simulink model "MySusp_TopMount_RTW"  (Simulink 10.3)
settings: Solver=ode1  StartTime=0.0  StopTime=inf  FixedStep=0.001  RelTol=1e-3
PreLoadFcn:
  | vehicle = 'Car'; if ~length(which('cmself')), cmenv; end
  | MySusp_TopMount_RTW_params
InitFcn:
  | vehicle = 'Car'; if ~length(which('cmself')), cmenv; end
  | MySusp_TopMount_RTW_bus
undefined symbols (not defined in the file or in its folder): cTM, dTM, mTM
Description:
  | CarMaker Plug-in Model Target
settings Model: Creator=ml  ModifiedByFormat=IPG  LastModifiedBy=IPG  MultithreadedSim=on
settings DataIOCC: SaveFormat=Dataset  SignalLoggingSaveFormat=Dataset  ReturnWorkspaceOutputs=on
settings OptimizationCC: ExpressionDepthLimit=128  LifeSpan=auto
settings DebuggingCC: UnderspecifiedInitializationDetection=Simplified  MergeDetectMultiDrivingBlocksExec=error  FcnCallInpInsideContextMsg=error  StateNameClashWarn=none  SFUnexpectedBacktrackingDiag=error  SFNoUnconditionalDefaultTransitionDiag=error  SFExecutionAtInitializationDiag=warning  ArithmeticOperatorsInVariantConditions=error
settings HardwareCC: ProdBitPerPointer=64  ProdBitPerSizeT=64  ProdBitPerPtrDiffT=64  ProdLargestAtomicFloat=Float  ProdIntDivRoundTo=Zero  ProdEndianess=LittleEndian  ProdWordSize=64  ProdHWDeviceType=Intel->x86-64 (Windows64)
settings ModelReferenceCC: PropagateSignalLabelsOutOfModel=on
settings SFSimCC: SimUseLocalCustomCode=on  CustomCodeUndefinedFunction=FilterOut
settings RTWCC: Description=CarMaker Plug-in Model Target  SystemTargetFile=CarMaker.tlc  TemplateMakefile=CarMaker_unix-win64.tmf  RTWUseLocalCustomCode=on
settings CodeAppCC: MaxIdLength=127  StateflowObjectComments=off
settings STFCustomTargetCC: TargetLangStandard=C99 (ISO)  CombineOutputUpdateFcns=on  CodeInterfacePackaging=Reusable function  GRTInterface=off  GenerateAllocFcn=on  SystemTargetFile=CarMaker.tlc
settings GRTTargetCC: TargetLangStandard=C99 (ISO)  ParMdlRefBuildCompliant=off  CompOptLevelCompliant=off  ConcurrentExecutionCompliant=off  CombineOutputUpdateFcns=on  MatFileLogging=off  CodeInterfacePackaging=Reusable function  CPPClassGenCompliant=off  GRTInterface=off  GenerateAllocFcn=on  UseToolchainInfoCompliant=off
settings CustomProperty: DataType=string
settings EnumStrPairs: String=Car
settings ConfigComp: CovMetricSettings=dwe  CovSaveCumulativeToWorkspaceVar=off  CovSaveSingleToWorkspaceVar=off  CovExternalEMLEnable=on

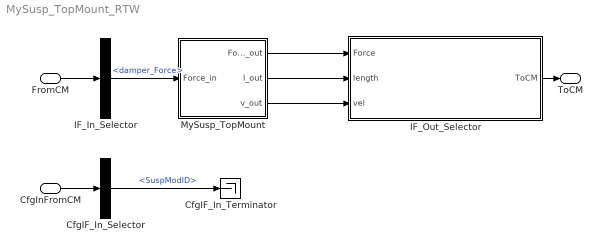
== system MySusp_TopMount_RTW ==
  FromCM : Inport  OutDataTypeStr=Bus: cmSusp_TopMountIn
  CfgInFromCM : Inport  Port=2  OutDataTypeStr=Bus: cmSusp_TopMountCfgIn
  CfgIF_In_Selector : BusSelector  OutputSignals=SuspModID
  CfgIF_In_Terminator : Terminator
  IF_In_Selector : BusSelector  OutputSignals=damper_Force
  IF_Out_Selector : Subsystem  mask(Signal Selection){}
      mask help: Signal Selection Block
      settings: OpenFcn=cmSignalSelect('SignalSelection_CB',gcb)
  MySusp_TopMount : Subsystem
  ToCM : Outport  OutDataTypeStr=Bus: cmSusp_TopMountOut
  wires:
  FromCM/1 -> IF_In_Selector/1
  IF_In_Selector/1 -> MySusp_TopMount/1(Force_in)  "<damper_Force>"
  IF_Out_Selector/1(ToCM) -> ToCM/1
  CfgInFromCM/1 -> CfgIF_In_Selector/1
  CfgIF_In_Selector/1 -> CfgIF_In_Terminator/1  "<SuspModID>"
  MySusp_TopMount/1(Force_out) -> IF_Out_Selector/1(Force)
  MySusp_TopMount/2(l_out) -> IF_Out_Selector/2(length)
  MySusp_TopMount/3(v_out) -> IF_Out_Selector/3(vel)

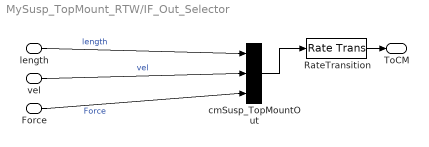
== system MySusp_TopMount_RTW/IF_Out_Selector ==
  Force : Inport
  length : Inport  Port=2
  vel : Inport  Port=3
  RateTransition : RateTransition  OutPortSampleTime=str2num(get_param(bdroot,'FixedStep'))
  cmSusp_TopMountOut : BusCreator  Inputs=3
  ToCM : Outport
  wires:
  RateTransition/1 -> ToCM/1
  cmSusp_TopMountOut/1 -> RateTransition/1
  length/1 -> cmSusp_TopMountOut/1  "length"
  Force/1 -> cmSusp_TopMountOut/3  "Force"
  vel/1 -> cmSusp_TopMountOut/2  "vel"

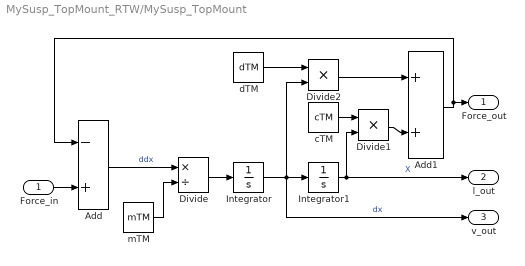
== system MySusp_TopMount_RTW/MySusp_TopMount ==
  Force_in : Inport
  Add : Sum  Inputs=-+
  Add1 : Sum
  Divide : Product  Inputs=*/
  Divide1 : Product  Inputs=**
  Divide2 : Product  Inputs=**
  Integrator : Integrator
  Integrator1 : Integrator
  cTM : Constant  Value=cTM
  dTM : Constant  Value=dTM
  mTM : Constant  Value=mTM
  Force_out : Outport  VectorParamsAs1DForOutWhenUnconnected=off
  l_out : Outport  Port=2  VectorParamsAs1DForOutWhenUnconnected=off
  v_out : Outport  Port=3  VectorParamsAs1DForOutWhenUnconnected=off
  wires:
  Integrator/1 -> Divide2/2, v_out/1, Integrator1/1  "dx"
  Integrator1/1 -> l_out/1, Divide1/2  "X"
  mTM/1 -> Divide/2
  Add/1 -> Divide/1  "ddx"
  Divide/1 -> Integrator/1
  cTM/1 -> Divide1/1
  dTM/1 -> Divide2/1
  Divide2/1 -> Add1/1
  Divide1/1 -> Add1/2
  Add1/1 -> Add/1, Force_out/1
  Force_in/1 -> Add/2
